simulink model "fsm_abstraction"  (Simulink 8.9)
settings: Solver=ode4  StartTime=0.0  StopTime=10  FixedStep=.1  RelTol=1e-3  EnableMultiTasking=on
settings Model: SuppressorTable=22 serialization::archive 11 0 6 0 0 0 0 0  Creator=elliocm  LastModifiedBy=dstaple
settings DataIOCC: SignalLoggingSaveFormat=Dataset
settings OptimizationCC: ExpressionDepthLimit=2147483647
settings DebuggingCC: SolverPrmCheckMsg=warning  FcnCallInpInsideContextMsg=error  AllowSymbolicDim=off
settings GRTTargetCC: CombineOutputUpdateFcns=on  GRTInterface=off

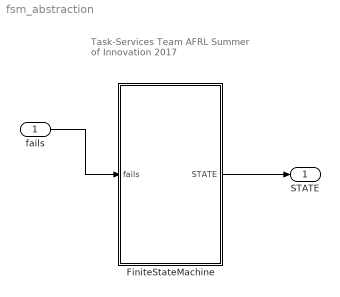
== system fsm_abstraction ==
  note: Task-Services Team
      | AFRL Summer of Innovation 2017
  fails : Inport  OutDataTypeStr=boolean
  FiniteStateMachine : Subsystem
  STATE : Outport
  wires:
  fails/1 -> FiniteStateMachine/1(fails)
  FiniteStateMachine/1(STATE) -> STATE/1

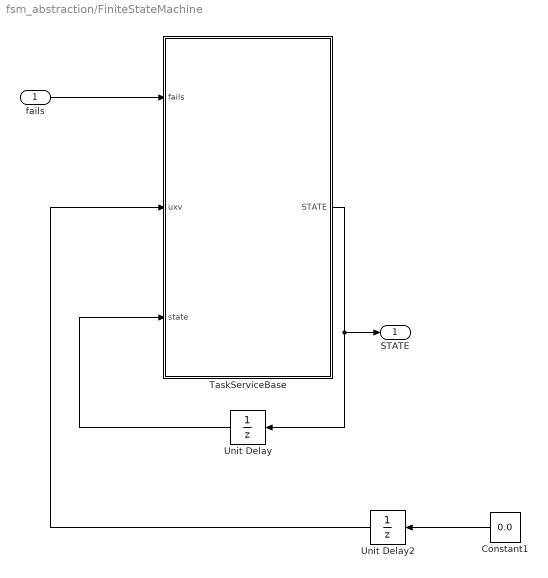
== system fsm_abstraction/FiniteStateMachine ==
  fails : Inport
  Constant1 : Constant  Value=0.0
  TaskServiceBase : Subsystem
  Unit Delay : UnitDelay  SampleTime=-1
  Unit Delay2 : UnitDelay  InitialCondition=1  SampleTime=-1
  STATE : Outport
  wires:
  TaskServiceBase/1(STATE) -> Unit Delay/1, STATE/1
  fails/1 -> TaskServiceBase/1(fails)
  Unit Delay/1 -> TaskServiceBase/3(state)
  Unit Delay2/1 -> TaskServiceBase/2(uxv)
  Constant1/1 -> Unit Delay2/1

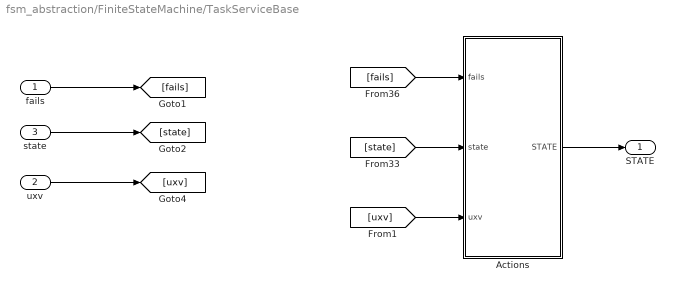
== system fsm_abstraction/FiniteStateMachine/TaskServiceBase ==
  fails : Inport
  uxv : Inport  Port=2
  state : Inport  Port=3
  Actions : Subsystem
  STATE : Outport
  wires:
  Actions/1(STATE) -> STATE/1
  [state] -> Actions/2(state)
  [fails] -> Actions/1(fails)
  [uxv] -> Actions/3(uxv)
  fails/1 -> [fails]
  state/1 -> [state]
  uxv/1 -> [uxv]

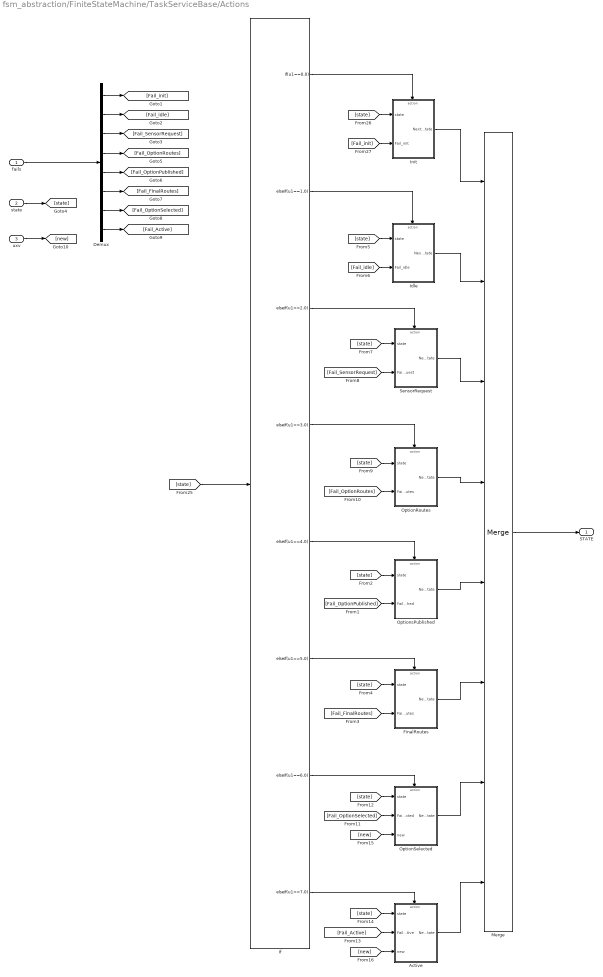
== system fsm_abstraction/FiniteStateMachine/TaskServiceBase/Actions ==
  fails : Inport
  state : Inport  Port=2
  uxv : Inport  Port=3
  Active : Subsystem
  Demux : Demux  Outputs=8
  FinalRoutes : Subsystem
  Idle : Subsystem
  If : If  IfExpression=u1==0.0  ElseIfExpressions=u1==1.0, u1==2.0, u1==3.0, u1==4.0, u1==5.0, u1==6.0, u1==7.0  ShowElse=off
  Init : Subsystem
  Merge : Merge  Inputs=8
  OptionRoutes : Subsystem
  OptionSelected : Subsystem
  OptionsPublished : Subsystem
  SensorRequest : Subsystem
  STATE : Outport
  wires:
  [state] -> If/1
  [state] -> Init/1(state)
  Merge/1 -> STATE/1
  Init/1(NextState) -> Merge/1
  If/2 -> Idle/Action
  If/4 -> OptionRoutes/Action
  If/1 -> Init/Action
  [Fail_init] -> Init/2(Fail_init)
  fails/1 -> Demux/1
  state/1 -> [state]
  OptionsPublished/1(NextState) -> Merge/5
  If/5 -> OptionsPublished/Action
  FinalRoutes/1(NextState) -> Merge/6
  If/6 -> FinalRoutes/Action
  If/7 -> OptionSelected/Action
  Active/1(NextState) -> Merge/8
  If/8 -> Active/Action
  [state] -> Idle/1(state)
  [Fail_idle] -> Idle/2(Fail_idle)
  Idle/1(NextState) -> Merge/2
  [state] -> SensorRequest/1(state)
  [Fail_SensorRequest] -> SensorRequest/2(Fail_SensorRequest)
  If/3 -> SensorRequest/Action
  SensorRequest/1(NextState) -> Merge/3
  [state] -> OptionRoutes/1(state)
  [Fail_OptionRoutes] -> OptionRoutes/2(Fail_OptionRoutes)
  OptionRoutes/1(NextState) -> Merge/4
  [state] -> OptionsPublished/1(state)
  [Fail_OptionPublished] -> OptionsPublished/2(Fail_OptionsPublished)
  [state] -> FinalRoutes/1(state)
  [Fail_FinalRoutes] -> FinalRoutes/2(Fail_FinalRoutes)
  [state] -> OptionSelected/1(state)
  [Fail_OptionSelected] -> OptionSelected/2(Fail_OptionSelected)
  OptionSelected/1(NextState) -> Merge/7
  [state] -> Active/1(state)
  [Fail_Active] -> Active/2(Fail_Active)
  Demux/1 -> [Fail_init]
  Demux/2 -> [Fail_idle]
  Demux/3 -> [Fail_SensorRequest]
  Demux/4 -> [Fail_OptionRoutes]
  Demux/5 -> [Fail_OptionPublished]
  Demux/6 -> [Fail_FinalRoutes]
  Demux/7 -> [Fail_OptionSelected]
  Demux/8 -> [Fail_Active]
  [new] -> OptionSelected/3(new)
  [new] -> Active/3(new)
  uxv/1 -> [new]

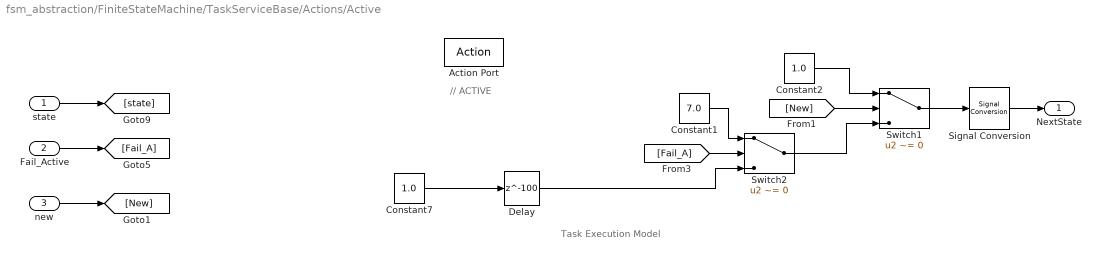
== system fsm_abstraction/FiniteStateMachine/TaskServiceBase/Actions/Active ==
  note: // ACTIVE
  note: Task Execution Model
  state : Inport
  Fail_Active : Inport  Port=2
  new : Inport  Port=3
  Action Port : ActionPort  ActionType=elseif
  Constant1 : Constant  Value=7.0
  Constant2 : Constant  Value=1.0
  Constant7 : Constant  Value=1.0
  Delay : Delay  DelayLength=100
  Signal Conversion : SignalConversion  OverrideOpt=off
  Switch1 : Switch  Criteria=u2 ~= 0
  Switch2 : Switch  Criteria=u2 ~= 0
  NextState : Outport
  wires:
  state/1 -> [state]
  Fail_Active/1 -> [Fail_A]
  Constant7/1 -> Delay/1
  [Fail_A] -> Switch2/2
  Constant1/1 -> Switch2/1
  Delay/1 -> Switch2/3
  Signal Conversion/1 -> NextState/1
  [New] -> Switch1/2
  Constant2/1 -> Switch1/1
  Switch1/1 -> Signal Conversion/1
  Switch2/1 -> Switch1/3
  new/1 -> [New]

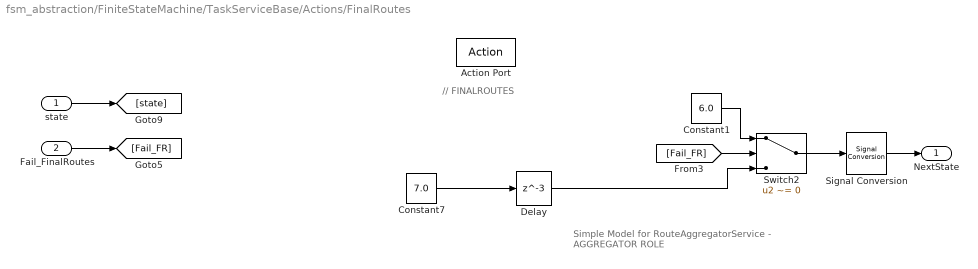
== system fsm_abstraction/FiniteStateMachine/TaskServiceBase/Actions/FinalRoutes ==
  note: Simple Model for
      | RouteAggregatorService - AGGREGATOR ROLE
  note: // FINALROUTES
  state : Inport
  Fail_FinalRoutes : Inport  Port=2
  Action Port : ActionPort  ActionType=elseif
  Constant1 : Constant  Value=6.0
  Constant7 : Constant  Value=7.0
  Delay : Delay  DelayLength=3
  Signal Conversion : SignalConversion  OverrideOpt=off
  Switch2 : Switch  Criteria=u2 ~= 0
  NextState : Outport
  wires:
  Signal Conversion/1 -> NextState/1
  Switch2/1 -> Signal Conversion/1
  Delay/1 -> Switch2/3
  Constant1/1 -> Switch2/1
  [Fail_FR] -> Switch2/2
  Constant7/1 -> Delay/1
  Fail_FinalRoutes/1 -> [Fail_FR]
  state/1 -> [state]

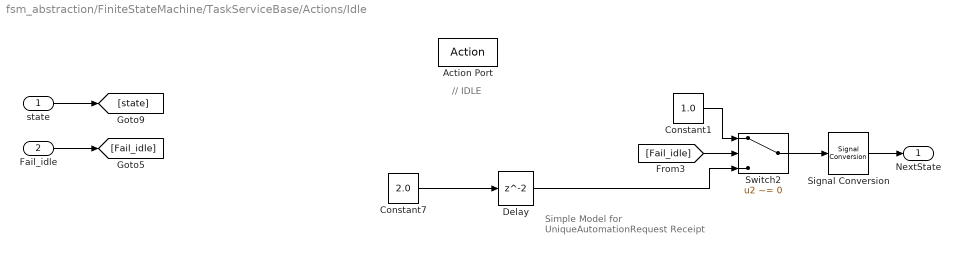
== system fsm_abstraction/FiniteStateMachine/TaskServiceBase/Actions/Idle ==
  note: Simple Model for
      | UniqueAutomationRequest Receipt
  note: // IDLE
  state : Inport
  Fail_idle : Inport  Port=2
  Action Port : ActionPort  ActionType=elseif
  Constant1 : Constant  Value=1.0
  Constant7 : Constant  Value=2.0
  Delay : Delay
  Signal Conversion : SignalConversion  OverrideOpt=off
  Switch2 : Switch  Criteria=u2 ~= 0
  NextState : Outport
  wires:
  state/1 -> [state]
  Fail_idle/1 -> [Fail_idle]
  Constant7/1 -> Delay/1
  [Fail_idle] -> Switch2/2
  Constant1/1 -> Switch2/1
  Delay/1 -> Switch2/3
  Switch2/1 -> Signal Conversion/1
  Signal Conversion/1 -> NextState/1

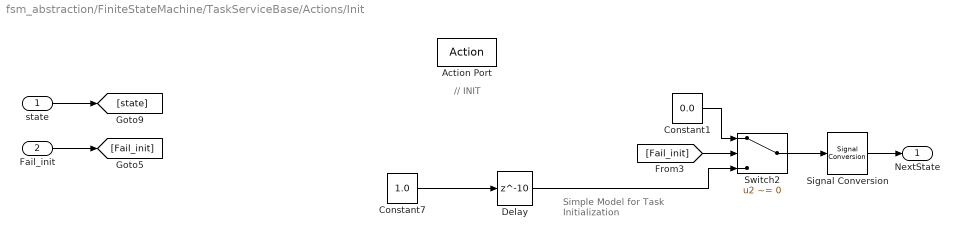
== system fsm_abstraction/FiniteStateMachine/TaskServiceBase/Actions/Init ==
  note: Simple Model
      | for Task Initialization
  note: // INIT
  state : Inport
  Fail_init : Inport  Port=2
  Action Port : ActionPort  ActionType=then
  Constant1 : Constant  Value=0.0
  Constant7 : Constant  Value=1.0
  Delay : Delay  DelayLength=10
  Signal Conversion : SignalConversion  OverrideOpt=off
  Switch2 : Switch  Criteria=u2 ~= 0
  NextState : Outport
  wires:
  state/1 -> [state]
  Fail_init/1 -> [Fail_init]
  Constant7/1 -> Delay/1
  [Fail_init] -> Switch2/2
  Constant1/1 -> Switch2/1
  Delay/1 -> Switch2/3
  Switch2/1 -> Signal Conversion/1
  Signal Conversion/1 -> NextState/1

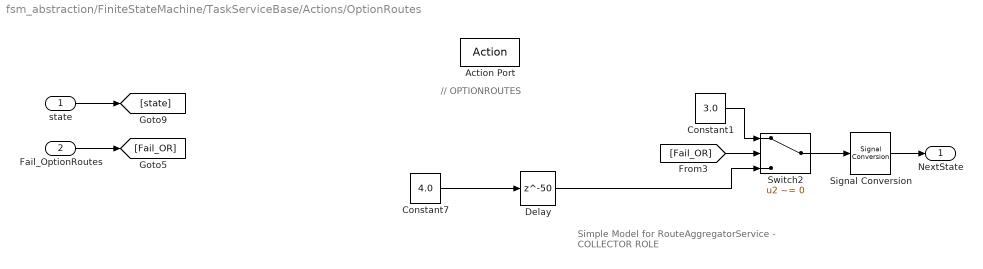
== system fsm_abstraction/FiniteStateMachine/TaskServiceBase/Actions/OptionRoutes ==
  note: Simple Model for
      | RouteAggregatorService - COLLECTOR ROLE
  note: // OPTIONROUTES
  state : Inport
  Fail_OptionRoutes : Inport  Port=2
  Action Port : ActionPort  ActionType=elseif
  Constant1 : Constant  Value=3.0
  Constant7 : Constant  Value=4.0
  Delay : Delay  DelayLength=50
  Signal Conversion : SignalConversion  OverrideOpt=off
  Switch2 : Switch  Criteria=u2 ~= 0
  NextState : Outport
  wires:
  Signal Conversion/1 -> NextState/1
  Switch2/1 -> Signal Conversion/1
  Delay/1 -> Switch2/3
  Constant1/1 -> Switch2/1
  [Fail_OR] -> Switch2/2
  Constant7/1 -> Delay/1
  Fail_OptionRoutes/1 -> [Fail_OR]
  state/1 -> [state]

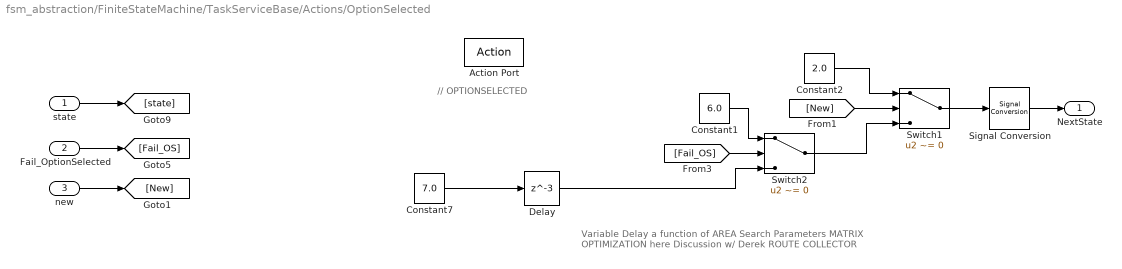
== system fsm_abstraction/FiniteStateMachine/TaskServiceBase/Actions/OptionSelected ==
  note: // OPTIONSELECTED
  note: Variable Delay a function of AREA Search Parameters
      | MATRIX OPTIMIZATION here
      | Discussion w/ Derek
      | ROUTE COLLECTOR
  state : Inport
  Fail_OptionSelected : Inport  Port=2
  new : Inport  Port=3
  Action Port : ActionPort  ActionType=elseif
  Constant1 : Constant  Value=6.0
  Constant2 : Constant  Value=2.0
  Constant7 : Constant  Value=7.0
  Delay : Delay  DelayLength=3
  Signal Conversion : SignalConversion  OverrideOpt=off
  Switch1 : Switch  Criteria=u2 ~= 0
  Switch2 : Switch  Criteria=u2 ~= 0
  NextState : Outport
  wires:
  state/1 -> [state]
  Fail_OptionSelected/1 -> [Fail_OS]
  Constant7/1 -> Delay/1
  [Fail_OS] -> Switch2/2
  Constant1/1 -> Switch2/1
  Delay/1 -> Switch2/3
  Signal Conversion/1 -> NextState/1
  [New] -> Switch1/2
  Constant2/1 -> Switch1/1
  Switch1/1 -> Signal Conversion/1
  Switch2/1 -> Switch1/3
  new/1 -> [New]

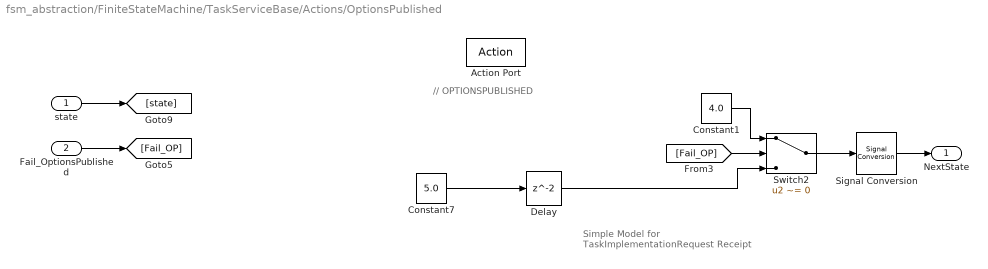
== system fsm_abstraction/FiniteStateMachine/TaskServiceBase/Actions/OptionsPublished ==
  note: // OPTIONSPUBLISHED
  note: Simple Model for
      | TaskImplementationRequest Receipt
  state : Inport
  Fail_OptionsPublished : Inport  Port=2
  Action Port : ActionPort  ActionType=elseif
  Constant1 : Constant  Value=4.0
  Constant7 : Constant  Value=5.0
  Delay : Delay
  Signal Conversion : SignalConversion  OverrideOpt=off
  Switch2 : Switch  Criteria=u2 ~= 0
  NextState : Outport
  wires:
  state/1 -> [state]
  Fail_OptionsPublished/1 -> [Fail_OP]
  Constant7/1 -> Delay/1
  [Fail_OP] -> Switch2/2
  Constant1/1 -> Switch2/1
  Delay/1 -> Switch2/3
  Switch2/1 -> Signal Conversion/1
  Signal Conversion/1 -> NextState/1

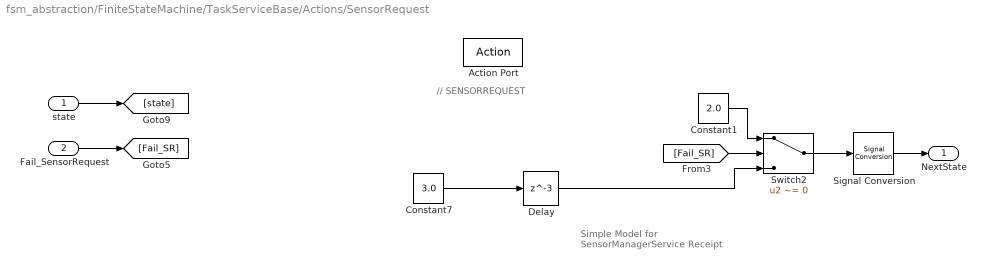
== system fsm_abstraction/FiniteStateMachine/TaskServiceBase/Actions/SensorRequest ==
  note: // SENSORREQUEST
  note: Simple Model for
      | SensorManagerService Receipt
  state : Inport
  Fail_SensorRequest : Inport  Port=2
  Action Port : ActionPort  ActionType=elseif
  Constant1 : Constant  Value=2.0
  Constant7 : Constant  Value=3.0
  Delay : Delay  DelayLength=3
  Signal Conversion : SignalConversion  OverrideOpt=off
  Switch2 : Switch  Criteria=u2 ~= 0
  NextState : Outport
  wires:
  state/1 -> [state]
  Fail_SensorRequest/1 -> [Fail_SR]
  Constant7/1 -> Delay/1
  [Fail_SR] -> Switch2/2
  Constant1/1 -> Switch2/1
  Delay/1 -> Switch2/3
  Switch2/1 -> Signal Conversion/1
  Signal Conversion/1 -> NextState/1
